simulink model "FMU_torque_vectoring4"  (R2023b)
settings: Solver=VariableStepAuto  StartTime=0.0  StopTime=50  RelTol=1e-3
values from neighbouring files (symbols this model uses):
  g = 9.8    [SetVehicleParameters.m]    (also in SetVehicleParameters2.m; SetVehicleParameters4.m; SetVehicleParameters5.m; SetVehicleParameters6.m)
  gearRatio = 7    [SetVehicleParameters2.m]    (also in SetVehicleParameters4.m; SetVehicleParameters5.m; SetVehicleParameters6.m)
  L = Lf + Lr    (= 3)    [SetVehicleParameters.m]    (also in SetVehicleParameters2.m = 2; SetVehicleParameters4.m = 2; SetVehicleParameters5.m = 2; SetVehicleParameters6.m = 2)
  Lr = 1.6    [SetVehicleParameters.m]    (also in SetVehicleParameters2.m = 0.5; SetVehicleParameters4.m = 0.5; SetVehicleParameters5.m = 0.5; SetVehicleParameters6.m = 0.5)
  rearTrackWidth = 1.4    [SetVehicleParameters.m]    (also in SetVehicleParameters2.m = 1; SetVehicleParameters4.m = 1; SetVehicleParameters5.m = 1; SetVehicleParameters6.m = 1)
  wheelRadius = 0.28    [SetVehicleParameters2.m]
libraries: commblkintrlv2 x1, vehdynlibviscommon x1, SignalEditorBlockLib x1, matrix_library x1, slpidlib x1
settings Model: Creator=denoc  LastModifiedBy=denoc

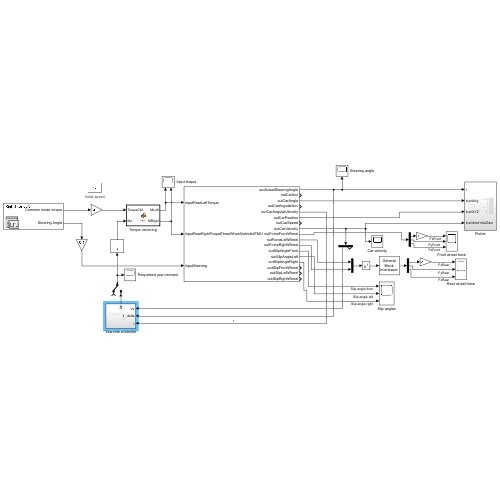
[thumbnail: Simulink's stored preview of the top-level diagram]
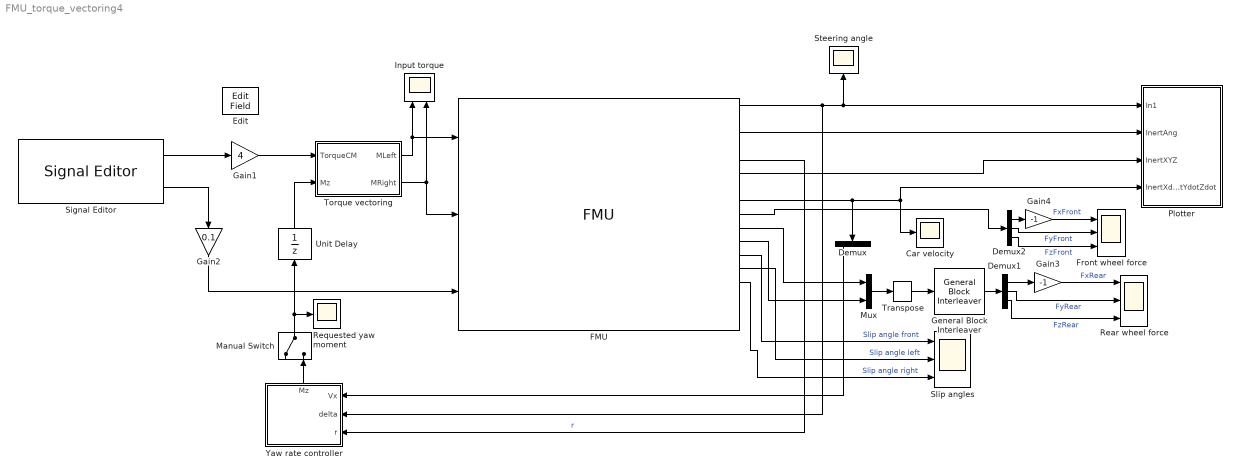
== system FMU_torque_vectoring4 ==
  Car velocity : Scope
  Demux : Demux  Outputs=2
  Demux1 : Demux  Outputs=3
  Demux2 : Demux  Outputs=3
  Edit : EditField  LabelPosition=Hide  ShowInitialText=on  Alignment=Center
      settings: AttributesFormatString=Initial speed
  FMU : FMU  FMUName=ThreeWheelVehicle2FMU.fmu  FMUMode=ModelExchange  FMUInitializeEnumObject=off  FMUCachedDialogLayout="{\"Geometry\":[738,126,689,534],\"ParameterColumnsWidthConfig\":\"{\\\"columns\\\":[{\\\"name\\\":\\\"Parameter\\\",\\\"width\\\":253},{\\\"name\\\":\\\"Value\\\",\\\"width\\\":171},{\\\"name\\\":\\\"Unit\\\",\\\"width\\\":156},{\\\"name\\\":\\\"Description\\\",\\\"width\\\":238}]}\",\"InputColumnsWidthConfig\":[],\"OutputColumnsWidthConfig\":\"{\\\"columns\\\":[{\\\"name\\\":\\\"Name\\\",\\\"width\\\":248},{\\\"name\\\":\\\"Visibility\\\",\\\"width\\\":79},{\\\"name\\\":\\\"Start\\\",\\\"width\\\":52},{\\\"name\\\":\\\"Unit\\\",\\\"width\\\":49},{\\\"name\\\":\\\"Type Object\\\",\\\"width\\\":107}]}\"}"  airResistanceLongitudinal=struct('r',[0.0,1.0],'rho',1.18)  backLength=Lr  body2=struct('I',1e-08,'m',0.1)  c_rollF=rollResF  c_rollL=rollResL  c_rollR=rollResR  dragCoef=dragCoeff  front=struct('r',[0.0],'width',0.2)  front2=struct('r',[1e-10,0.0])  frontLength=Lf  frontTrail=struct('r',[0.0,-0.1])  frontWheel=struct('diameter',0.1,'r',[0.0,1.0],'v0_roll',0.1)  g=g  gearRatio=gearRatio  inertiaBody=Izz  inertiaWheelF=inertiaF  inertiaWheelL=inertiaL  inertiaWheelR=inertiaR  mass=mass  massCenterZ=h  muAF=muAF  muAL=muAL  muAR=muAR  muSF=muSF  muSL=muSL  muSR=muSR  neg=struct('k',-1.0)  neg2=struct('k',-1.0)  planarWorld=struct('constantGravity',[0.0,0.0],'defaultFrameDiameterFraction',40.0,'defaultN_to_m',1000.0,'defaultNm_to_m',1000.0,'defaultSpecularCoefficient',0.7,'defaultWidthFraction',20.0,'defaultZPosition',0.0,'gravityArrowTail',[0.0,0.0],'nominalLength',1.0)  positionPhi=struct('f_crit',50.0)  rear=struct('r',[0.0],'width',0.2)  rearLeft=struct('r',[0,0.0])  rearLeftWheel=struct('diameter',0.1,'r',[0.0,1.0],'v0_roll',0.1)  rearRight=struct('r',[0,0.0])  rearRightWheel=struct('diameter',0.1,'r',[0.0,1.0],'v0_roll',0.1)  sAdF=sAdF  sAdL=sAdL  sAdR=sAdR  sSlF=sSlF  sSlL=sSlL  sSlR=sSlR  speedStart=12  turnRadiusMAX=1000.0  vAdF=vAdF  vAdL=vAdL  vAdR=vAdR  vSlF=vSlF  vSlL=vSlL  vSlR=vSlR  vehicleFrontArea=1.5  vehicleWidth=rearTrackWidth  wheelRadiusF=wheelRadiusF  wheelRadiusL=wheelRadiusL  wheelRadiusR=wheelRadiusR  body_sphere_shapeType=sphere  body2_sphere_shapeType=sphere  front_cylinder_shapeType=cylinder  front2_cylinder_shapeType=cylinder  frontTrail_cylinder_shapeType=cylinder  frontWheel_cylinder_shapeType=cylinder  frontWheel_rim1_shapeType=cylinder  frontWheel_rim2_shapeType=cylinder  planarWorld_label1=x  planarWorld_label2=y  rear_cylinder_shapeType=cylinder  rearLeft_cylinder_shapeType=cylinder  rearLeftWheel_cylinder_shapeType=cylinder  rearLeftWheel_rim1_shapeType=cylinder  rearLeftWheel_rim2_shapeType=cylinder  rearRight_cylinder_shapeType=cylinder  rearRightWheel_cylinder_shapeType=cylinder  rearRightWheel_rim1_shapeType=cylinder  rearRightWheel_rim2_shapeType=cylinder  revolute_cylinder_shapeType=cylinder  mask(ThreeWheelVehicle2FMU [Model Exchange, v2.0]){}
      settings: MultithreadedSim=off
      mask Display:
      | disp('ThreeWheelVehicle2FMU');
      | port_label('output',1,'outActualSteeringAngle');
      | port_label('output',2,'outCarAcc');
      | port_label('output',3,'outCarAngle');
      | port_label('output',4,'outCarAngularAcc');
      | port_label('output',5,'outCarAngularVelocity');
      | port_label('output',6,'outCarPosition');
      | port_label('output',7,'outCarSpeed');
      | port_label('output',8,'outCarVelocity');
      | port_label('output',9,'outForceFrontWheel');
      | port_label('output',10,'outForceLeftWheel');
      | port_label('output',11,'outForceRightWheel');
      | port_label('output',12,'outSlipAngleFront');
      | port_label('output',13,'outSlipAngleLeft');
      | port_label('output',14,'outSlipAngleRight');
      | port_label('output',15,'outSlipFrontWheel');
      | port_label('output',16,'outSlipLeftWheel');
      | port_label('output',17,'outSlipRightWheel');
      | port_label('input',1,'inputRearLeftTorque');
      | port_label('input',2,'inputRearRightTorque');
      | port_label('input',3,'inputSteering');
  Front wheel force : Scope  NumInputPorts=3
  Gain1 : Gain  Gain=4
  Gain2 : Gain  Gain=0.1
  Gain3 : Gain  Gain=-1
  Gain4 : Gain  Gain=-1
  General Block Interleaver : commblkintrlv2/General Block Interleaver  StatePerturbationForJacobian=1.0e-05  permutationVectorSource=Dialog  elements=[1;4;2;5;3;6]
  Input torque : Scope  NumInputPorts=2
  Manual Switch : ManualSwitch
  Mux : Mux  Inputs=2
  Plotter : Subsystem
  Rear wheel force : Scope  NumInputPorts=3
  Requested yaw moment : Scope
  Signal Editor : SignalEditorBlockLib/Signal Editor  FileName=signals.mat  ActiveScenario=RightThenLeft  ActiveSignal=Steering Angle  IsBus=off  OutputBusObjectStr=Bus: BusObject  SampleTime=0  ZeroCross=off  OutputAfterFinalValue=Holding final value  Unit=inherit  PreserveSignalName=on  ApplySigPropsToAllScenarios=on  ApplySigPropsToAllSignals=on
  Slip angles : Scope  NumInputPorts=3
  Steering angle : Scope
  Torque vectoring : MATLAB Function  TreatAsAtomicUnit=on
  Transpose : matrix_library/Transpose
  Unit Delay : UnitDelay  SampleTime=0.001  HasFrameUpgradeWarning=on
  Yaw rate controller : Subsystem
      settings: PortSchema="{\"entries\":[{\"content\":{\"sides\":[{\"content\":{},\"type\":\"ConnectorPlacement.EquallySpacedRectSide\",\"uuid\":\"857998bb-17b2-4c26-a88e-7a272ab33241\"},{\"content\":{\"connectorIds\":[\"In1\",\"In2\",\"In3\"],\"side\":\"RIGHT\"},\"type\":\"ConnectorPlacement.EquallySpacedRectSide\",\"uuid\":\"e6bac797-4ab7-4d5a-9049-404e840be7e3\"},{\"content\":{\"connectorIds\":[\"Out1\"],\"side\":\"TOP\"},\"type\":\"ConnectorPlacement.EquallySpacedRectSide\",\"uuid\":\"452e310b-aafe-4970-ab47-27f3c9e5aadb\"}]},\"type\":\"ConnectorPlacement.EquallySpacedConnector\",\"uuid\":\"c70c4af1-0cf8-460a-ae4f-0fb1bd9e22f3\"}],\"packageUris\":[\"http://schema.mathworks.com/mf0/Connector/R2020b\"],\"version\":\"1.0\"}"
  wires:
  Signal Editor/2 -> Gain2/1
  Signal Editor/1 -> Gain1/1
  Gain2/1 -> FMU/3
  FMU/3 -> Plotter/2(InertAng)
  FMU/6 -> Plotter/3(InertXYZ)
  FMU/8 -> Car velocity/1, Plotter/4(InertXdotYdotZdot), Demux/1
  Demux/1 -> Yaw rate controller/1(Vx)
  Yaw rate controller/1(Mz) -> Manual Switch/2
  Manual Switch/1 -> Requested yaw moment/1, Unit Delay/1
  Gain1/1 -> Torque vectoring/1(TorqueCM)
  Torque vectoring/1(MLeft) -> FMU/1, Input torque/1
  Torque vectoring/2(MRight) -> FMU/2, Input torque/2
  Unit Delay/1 -> Torque vectoring/2(Mz)
  FMU/5 -> Yaw rate controller/3(r)  "r"
  FMU/10 -> Mux/1
  FMU/11 -> Mux/2
  FMU/1 -> Yaw rate controller/2(delta), Steering angle/1, Plotter/1(In1)
  General Block Interleaver/1 -> Demux1/1
  Demux1/1 -> Gain3/1
  Demux1/2 -> Rear wheel force/2  "FyRear"
  Demux1/3 -> Rear wheel force/3  "FzRear"
  Mux/1 -> Transpose/1
  Transpose/1 -> General Block Interleaver/1
  Gain3/1 -> Rear wheel force/1  "FxRear"
  Demux2/1 -> Gain4/1
  Demux2/2 -> Front wheel force/2  "FyFront"
  Demux2/3 -> Front wheel force/3  "FzFront"
  FMU/9 -> Demux2/1
  Gain4/1 -> Front wheel force/1  "FxFront"
  FMU/12 -> Slip angles/1  "Slip angle front"
  FMU/13 -> Slip angles/2  "Slip angle left"
  FMU/14 -> Slip angles/3  "Slip angle right"

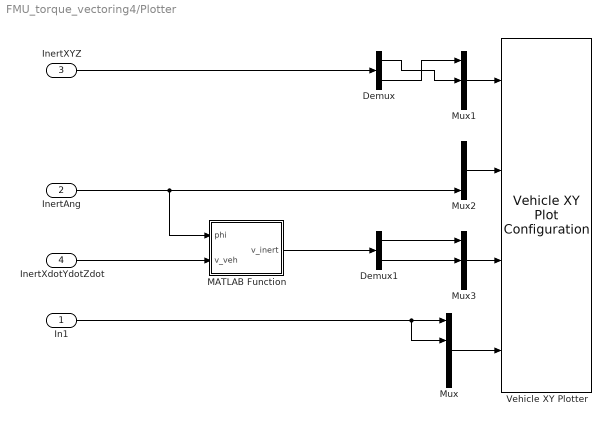
== system FMU_torque_vectoring4/Plotter ==
  In1 : Inport
  InertAng : Inport  Port=2
  InertXYZ : Inport  Port=3
  InertXdotYdotZdot : Inport  Port=4
  Demux : Demux  Outputs=2
  Demux1 : Demux  Outputs=2
  MATLAB Function : MATLAB Function  TreatAsAtomicUnit=on
  Mux : Mux
  Mux1 : Mux  Inputs=3
  Mux2 : Mux  Inputs=3
  Mux3 : Mux  Inputs=3
  Vehicle XY Plotter : vehdynlibviscommon/Vehicle XY Plot Configuration  extRef=off  extStats=off  extTireF=off  a=Lf  b=Lr  w=rearTrackWidth  figBorder=10  bufferSize=1024  velNorm=5  tireFNorm=1000  pltDT=.1
  wires:
  Mux/1 -> Vehicle XY Plotter/4
  Mux1/1 -> Vehicle XY Plotter/1
  Mux2/1 -> Vehicle XY Plotter/2
  InertAng/1 -> MATLAB Function/1(phi), Mux2/3
  InertXYZ/1 -> Demux/1
  Demux1/2 -> Mux3/2
  Demux1/1 -> Mux3/1
  Mux3/1 -> Vehicle XY Plotter/3
  Demux/2 -> Mux1/1
  Demux/1 -> Mux1/2
  In1/1 -> Mux/2, Mux/1
  InertXdotYdotZdot/1 -> MATLAB Function/2(v_veh)
  MATLAB Function/1(v_inert) -> Demux1/1

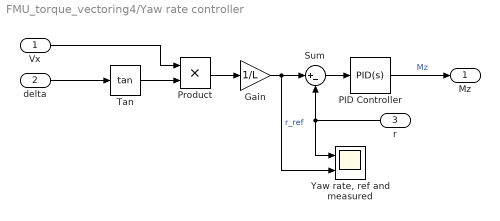
== system FMU_torque_vectoring4/Yaw rate controller ==
  Vx : Inport
  delta : Inport  Port=2
  r : Inport  Port=3
  Gain : Gain  Gain=1/L
  PID Controller : slpidlib/PID Controller  Controller=PID  Form=Parallel  TimeDomain=Continuous-time  UseExternalTs=off  SampleTime=-1  IntegratorMethod=Forward Euler  FilterMethod=Forward Euler  ControllerParametersSource=internal  P=700  I=180  UseKiTs=off  D=0  N=100  UseFilter=on  TunerSelectOption=Transfer Function Based (PID Tuner App)  InitialConditionSource=internal  InitialConditionForIntegrator=0  InitialConditionForFilter=0  DifferentiatorICPrevScaledInput=0  ExternalReset=none  TrackingMode=off  Kt=1  LimitOutput=off  SatLimitsSource=internal  UpperSaturationLimit=inf  LowerSaturationLimit=-inf  LinearizeAsGain=on  AntiWindupMode=none  Kb=1  LimitIntegrator=off  UpperIntegratorSaturationLimit=inf  LowerIntegratorSaturationLimit=-inf  POutMin=[]  POutMax=[]  IOutMin=[]  IOutMax=[]  DOutMin=[]  DOutMax=[]  NOutMin=[]  NOutMax=[]  SumOutMin=[]  SumOutMax=[]  SaturationOutMin=[]  SaturationOutMax=[]  PParamMin=[]  PParamMax=[]  IParamMin=[]  IParamMax=[]  DParamMin=[]  DParamMax=[]  NParamMin=[]  NParamMax=[]  KbParamMin=[]  KbParamMax=[]  KtParamMin=[]  KtParamMax=[]  KbOutMin=[]  KbOutMax=[]  KtOutMin=[]  KtOutMax=[]  IntegratorOutMin=[]  IntegratorOutMax=[]  FilterOutMin=[]  FilterOutMax=[]  SumI1OutMin=[]  SumI1OutMax=[]  SumI2OutMin=[]  SumI2OutMax=[]  SumI3OutMin=[]  SumI3OutMax=[]  SumI4OutMin=[]  SumI4OutMax=[]  SumDOutMin=[]  SumDOutMax=[]  DifferentiatorOutMin=[]  DifferentiatorOutMax=[]  FilterDiffOutCoefMin=[]  FilterDiffOutCoefMax=[]  ReciprocalOutMin=[]  ReciprocalOutMax=[]  SumDenOutMin=[]  SumDenOutMax=[]  SumNumOutMin=[]  SumNumOutMax=[]  DivideOutMin=[]  DivideOutMax=[]  UdiffTsProdOutMin=[]  UdiffTsProdOutMax=[]  NTsProdOutMin=[]  NTsProdOutMax=[]  UintegralTsProdOutMin=[]  UintegralTsProdOutMax=[]  UngainTsProdOutMin=[]  UngainTsProdOutMax=[]  ClampingZeroOutDataTypeStr=Inherit: Inherit via back propagation  ClampingZeroOutMin=[]  ClampingZeroOutMax=[]  FilterDenConstantOutDataTypeStr=Inherit: Inherit via back propagation  FilterDenConstantOutMin=[]  FilterDenConstantOutMax=[]  PCopyOutDataTypeStr=Inherit: Inherit via back propagation  PCopyOutMin=[]  PCopyOutMax=[]  NCopyOutDataTypeStr=Inherit: Inherit via back propagation  NCopyOutMin=[]  NCopyOutMax=[]  IntegratorContinuousStateAttributes=''  IntegratorStateMustResolveToSignalObject=off  IntegratorRTWStateStorageClass=Auto  FilterContinuousStateAttributes=''  FilterStateMustResolveToSignalObject=off  FilterRTWStateStorageClass=Auto  ParallelPVariant=InternalParameters  IdealPVariant=Disabled  IVariant=InternalParameters  DVariant=InternalParameters  IntegratorVariant=Continuous  SatVariant=Disabled  AWVariant=Passthrough  PCopyVariant=Disabled  TRVariant=Disabled  FdbkBlocksVariant=Forward  IdealPFdbkVariant=Disabled  SatFdbkVariant=Disabled  DerivativeFilterVariant=ContFilter  NVariant=InternalParameters  NCopyVariant=Disabled  FilterICVariant=InternalICsFilter  IntegratorICVariant=InternalICs  ExternalResetVariant=Disabled  TRSumVariant=Passthrough  SumFdbkVariant=Disabled  SumVariant=Sum_PID  TsampFilterVariant=InternalTs  TsampNgainVariant=Passthrough  TsampIntegralVariant=Disabled_SignalSpec  ExternalSaturationOutDataTypeStr=Inherit: Same as second input
  Product : Product
  Sum : Sum  Inputs=|+-
  Tan : Trigonometry  Operator=tan
  "Yaw rate, ref and measured" : Scope  NumInputPorts=2
  Mz : Outport
  wires:
  Gain/1 -> Sum/1, "Yaw rate, ref and measured"/2  "r_ref"
  PID Controller/1 -> Mz/1  "Mz"
  Sum/1 -> PID Controller/1
  r/1 -> Sum/2, "Yaw rate, ref and measured"/1
  Product/1 -> Gain/1
  Tan/1 -> Product/2
  delta/1 -> Tan/1
  Vx/1 -> Product/1

== matlab function FMU_torque_vectoring4/Torque vectoring ==
  data: TorqueCM input; Mz input; MLeft output; MRight output; gearRatio parameter; wheelRadius parameter; rearTrackWidth parameter
function [MLeft, MRight] = fcn(TorqueCM, Mz, gearRatio, wheelRadius, rearTrackWidth)

MDiff = wheelRadius * Mz / (gearRatio * rearTrackWidth);
MLeft = TorqueCM + MDiff;
MRight = TorqueCM - MDiff;

== matlab function FMU_torque_vectoring4/Plotter/MATLAB Function ==
  data: phi input; v_veh input; v_inert output
function v_inert  = fcn(phi, v_veh)

R = [cos(phi), -sin(phi); 
     sin(phi), cos(phi)];

v_inert = R * v_veh;
